simulink model "CrashAlgoSchnee_v2_analysis"  (R2020b)
settings: Solver=FixedStepAuto  StartTime=0.0  StopTime=inf  FixedStep=0.01  RelTol=1e-3
undefined symbols (not defined in the file or in its folder): magnitude
libraries: simulink x2
settings Model: Creator=snj7rt  LastModifiedBy=HNA3SI
settings DataIOCC: SaveOutput=off  SaveTime=off  ReturnWorkspaceOutputs=off
settings DebuggingCC: ArithmeticOperatorsInVariantConditions=warning
settings ModelReferenceCC: ModelReferenceNumInstancesAllowed=Single
settings SFSimCC: CustomCodeUndefinedFunction=UseInterfaceOnly
settings GRTTargetCC: CombineOutputUpdateFcns=off  MatFileLogging=off

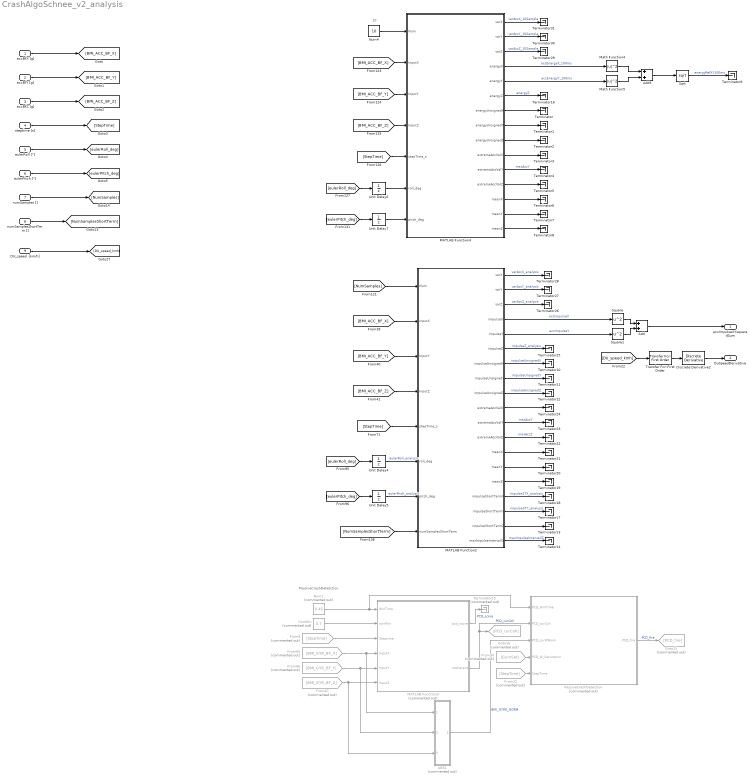
== system CrashAlgoSchnee_v2_analysis ==
  note: 10
  note: PassiveCrashDetetction
  accBfX [g] : Inport
  accBfY [g] : Inport  Port=2
  accBfZ [g] : Inport  Port=3
  steptime [s] : Inport  Port=4
  eulerRoll [°] : Inport  Port=5
  eulerPitch [°] : Inport  Port=6
  numSamples [] : Inport  Port=7
  numSamplesShortTerm [] : Inport  Port=8
  DU_speed  [km/h] : Inport  Port=9
  ABS1 : Subsystem  Commented=on
  Add : Sum
  Add3 : Sum
  CorrMin : Constant  Commented=on  Value=0.7
  Discrete Derivative2 : simulink/Discrete/Discrete Derivative  gainval=1.0  ICPrevScaledInput=0.0  OutMin=[]  OutMax=[]  OutDataType=fixdt(1, 16)  OutScaling=2^-10  DoSatur=off
  From12 : From  Commented=on  GotoTag=StepTime
  From30 : From  Commented=on  GotoTag=GyroSat
  From65 : From  Commented=on  GotoTag=BMI_GYR_BF_X
  From66 : From  Commented=on  GotoTag=BMI_GYR_BF_Y
  From67 : From  Commented=on  GotoTag=BMI_GYR_BF_Z
  From8 : From  Commented=on  GotoTag=StepTime
  Goto15 : Goto  Commented=on  GotoTag=PCD_fire
  Goto16 : Goto  Commented=on  GotoTag=PCD_curCoh
  MATLAB Function2 : MATLAB Function  TreatAsAtomicUnit=on
  MATLAB Function3 : MATLAB Function  Commented=on  TreatAsAtomicUnit=on
  MATLAB Function4 : MATLAB Function  TreatAsAtomicUnit=on
  Math Function4 : Math  Operator=magnitude^2  SignedPower=on  SaturateOnIntegerOverflow=on
  Math Function5 : Math  Operator=magnitude^2  SignedPower=on  SaturateOnIntegerOverflow=on
  Num1 : Constant  Commented=on  Value=0.45
  Num4 : Constant  Value=10
  PassiveCrashDetection : Stateflow chart  Commented=on  TreatAsAtomicUnit=on
  Sqrt : Sqrt  SaturateOnIntegerOverflow=on
  Square : Math  Operator=square  SignedPower=on  SaturateOnIntegerOverflow=on
  Square1 : Math  Operator=square  SignedPower=on  SaturateOnIntegerOverflow=on
  Terminator{,1..14,16..31} (31 alike) : Terminator
  Terminator15 : Terminator  Commented=on
  Transfer Fcn First Order : simulink/Discrete/Transfer Fcn First Order  PoleZ=0.995  ICPrevOutput=0.0  DoSatur=off
  Unit Delay{4..7} (4 alike) : UnitDelay  SampleTime=-1  HasFrameUpgradeWarning=on
  accImpulseXYsquaredSum : Outport
  DuSpeedDerivative : Outport  Port=2
  wires:
  [BMI_ACC_BF_X] -> MATLAB Function4/2(InputX)
  MATLAB Function4/3(varZ) -> Terminator29/1  "varAccZ_10Sample"
  Unit Delay7/1 -> MATLAB Function4/7(pitch_deg)
  MATLAB Function4/4(energyX) -> Math Function4/1  "accEnergyX_100ms"
  MATLAB Function4/5(energyY) -> Math Function5/1  "accEnergyY_100ms"
  MATLAB Function4/1(varX) -> Terminator31/1  "varAccX_10Sample"
  MATLAB Function4/2(varY) -> Terminator30/1  "varAccY_10Sample"
  [eulerRoll_deg] -> Unit Delay6/1
  Unit Delay6/1 -> MATLAB Function4/6(roll_deg)
  [eulerPitch_deg] -> Unit Delay7/1
  [BMI_ACC_BF_Z] -> MATLAB Function4/4(InputZ)
  Num4/1 -> MATLAB Function4/1(Num)
  [BMI_ACC_BF_Y] -> MATLAB Function4/3(InputY)
  [StepTime] -> MATLAB Function4/5(stepTime_s)
  accBfX [g]/1 -> [BMI_ACC_BF_X]
  accBfY [g]/1 -> [BMI_ACC_BF_Y]
  accBfZ [g]/1 -> [BMI_ACC_BF_Z]
  steptime [s]/1 -> [StepTime]
  eulerRoll [°]/1 -> [eulerRoll_deg]
  eulerPitch [°]/1 -> [eulerPitch_deg]
  [BMI_ACC_BF_X] -> MATLAB Function2/2(InputX)
  [StepTime] -> MATLAB Function2/5(stepTime_s)
  MATLAB Function2/17(impulseShortTermY) -> Terminator17/1  "impulseSTY_analysis"
  MATLAB Function2/7(impulseUnsignedX) -> Terminator10/1  "impulseUnsignedX"
  MATLAB Function2/19(maxImpulseIntervallZ) -> Terminator14/1  "maxImpulseIntervallZ"
  [NumSamplesShortTerm] -> MATLAB Function2/8(numSamplesShortTerm)
  [NumSamples] -> MATLAB Function2/1(Num)
  Unit Delay4/1 -> MATLAB Function2/6(roll_deg)  "eulerRoll_analysis"
  [eulerRoll_deg] -> Unit Delay4/1
  MATLAB Function2/8(impulseUnsignedY) -> Terminator11/1  "impulseUnsignedY"
  Unit Delay5/1 -> MATLAB Function2/7(pitch_deg)  "eulerPitch_analysis"
  [eulerPitch_deg] -> Unit Delay5/1
  MATLAB Function2/12(extremaAccValZ) -> Terminator22/1  "maxAccZ"
  MATLAB Function2/9(impulseUnsignedZ) -> Terminator12/1  "impulseUnsignedZ"
  MATLAB Function2/6(impulseZ) -> Terminator25/1  "impulseZ_analysis"
  MATLAB Function2/2(varY) -> Terminator27/1  "varAccY_analysis"
  MATLAB Function2/1(varX) -> Terminator28/1  "varAccX_analysis"
  MATLAB Function2/5(impulseY) -> Square1/1  "accImpulseY"
  [BMI_ACC_BF_Z] -> MATLAB Function2/4(InputZ)
  [BMI_ACC_BF_Y] -> MATLAB Function2/3(InputY)
  MATLAB Function2/4(impulseX) -> Square/1  "accImpulseX"
  MATLAB Function2/3(varZ) -> Terminator26/1  "varAccZ_analysis"
  MATLAB Function2/16(impulseShortTermX) -> Terminator18/1  "impulseSTX_analysis"
  MATLAB Function2/10(extremaAccValX) -> Terminator24/1
  MATLAB Function2/11(extremaAccValY) -> Terminator23/1  "maxAccY"
  MATLAB Function3/1(pcd_score) -> Terminator15/1  "PCD_score"
  From66/1 -> ABS1/2(In2), MATLAB Function3/5(InputY)
  From8/1 -> MATLAB Function3/3(Steptime)
  PassiveCrashDetection/1(PCD_fire) -> Goto15/1  "PCD_fire"
  From30/1 -> PassiveCrashDetection/4(PCD_W_Saturation)
  ABS1/1(Out1) -> PassiveCrashDetection/3(PCD_curWNorm)  "BMI_GYRO_NORM"
  From12/1 -> PassiveCrashDetection/5(StepTime)
  Num1/1 -> PassiveCrashDetection/1(PCD_WinTime), MATLAB Function3/1(WinTime)
  From65/1 -> ABS1/1(In1), MATLAB Function3/4(InputX)
  MATLAB Function3/2(ncoherent) -> Goto16/1, PassiveCrashDetection/2(PCD_curCoh)  "PCD_curCoh"
  From67/1 -> MATLAB Function3/6(InputZ), ABS1/3(In3)
  CorrMin/1 -> MATLAB Function3/2(corrMin)
  numSamples []/1 -> [NumSamples]
  numSamplesShortTerm []/1 -> [NumSamplesShortTerm]
  DU_speed  [km/h]/1 -> [DU_speed_kmh]
  MATLAB Function2/15(meanZ) -> Terminator19/1
  MATLAB Function2/14(meanY) -> Terminator20/1
  MATLAB Function2/13(meanX) -> Terminator21/1
  Math Function4/1 -> Add3/1
  Math Function5/1 -> Add3/2
  Add3/1 -> Sqrt/1
  Sqrt/1 -> Terminator9/1  "energyRefXY100ms"
  [DU_speed_kmh] -> Transfer Fcn First Order/1
  Discrete Derivative2/1 -> DuSpeedDerivative/1
  Transfer Fcn First Order/1 -> Discrete Derivative2/1
  MATLAB Function4/6(energyZ) -> Terminator16/1  "energyZ"
  MATLAB Function4/7(energyUnsignedX) -> Terminator/1
  MATLAB Function4/8(energyUnsignedY) -> Terminator1/1
  MATLAB Function4/9(energyUnsignedZ) -> Terminator2/1
  MATLAB Function4/10(extremaAccValX) -> Terminator3/1
  MATLAB Function4/11(extremaAccValY) -> Terminator4/1  "maxAccY"
  MATLAB Function4/12(extremaAccValZ) -> Terminator5/1
  MATLAB Function4/13(meanX) -> Terminator6/1
  MATLAB Function4/14(meanY) -> Terminator7/1
  MATLAB Function4/15(meanZ) -> Terminator8/1
  MATLAB Function2/18(impulseShortTermZ) -> Terminator13/1
  Square/1 -> Add/1
  Square1/1 -> Add/2
  Add/1 -> accImpulseXYsquaredSum/1

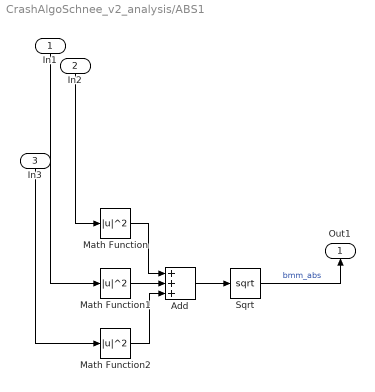
== system CrashAlgoSchnee_v2_analysis/ABS1 ==
  In1 : Inport
  In2 : Inport  Port=2
  In3 : Inport  Port=3
  Add : Sum  Inputs=+++
  Math Function : Math  Operator=magnitude^2  SignedPower=on  SaturateOnIntegerOverflow=on
  Math Function1 : Math  Operator=magnitude^2  SignedPower=on  SaturateOnIntegerOverflow=on
  Math Function2 : Math  Operator=magnitude^2  SignedPower=on  SaturateOnIntegerOverflow=on
  Sqrt : Sqrt  SaturateOnIntegerOverflow=on
  Out1 : Outport  VectorParamsAs1DForOutWhenUnconnected=off
  wires:
  In3/1 -> Math Function2/1
  In2/1 -> Math Function/1
  In1/1 -> Math Function1/1
  Math Function2/1 -> Add/3
  Add/1 -> Sqrt/1
  Math Function/1 -> Add/1
  Math Function1/1 -> Add/2
  Sqrt/1 -> Out1/1  "bmm_abs"

== matlab function CrashAlgoSchnee_v2_analysis/MATLAB Function4 ==
  data: Num input; InputX input; InputY input; InputZ input; varX output; varY output; varZ output; energyX output; energyY output; energyZ output; energyUnsignedX output; energyUnsignedY output; energyUnsignedZ output; stepTime_s input; extremaAccValX output; extremaAccValY output; roll_deg input; pitch_deg input; extremaAccValZ output; meanX output; meanY output; meanZ output
function [varX, varY, varZ, energyX, energyY, energyZ, ...
    energyUnsignedX, energyUnsignedY, energyUnsignedZ, ...
    extremaAccValX, extremaAccValY, extremaAccValZ, meanX, meanY, meanZ] = ...
    varPastNumSamples(Num, ...
    InputX, InputY, InputZ, stepTime_s, roll_deg, pitch_deg)

persistent ringBufX ringBufY ringBufZ i ringBufXgComp ringBufYgComp  
        
%% declaration only during first run!

if isempty(i)  
        ringBufX =ones(Num,1);
        ringBufY =ones(Num,1);
        ringBufYgComp =ones(Num,1);
        ringBufXgComp =ones(Num,1);
        ringBufZ =ones(Num,1);
        i = 1; 
end

ringBufX(i)= InputX;
ringBufY(i)= InputY;
ringBufYgComp(i)= InputY - sind(roll_deg);
ringBufXgComp(i)= InputX + sind(pitch_deg);
ringBufZ(i)= InputZ;

varX = var(ringBufX, 0);
varY = var(ringBufY, 0);
varZ = var(ringBufZ, 0);

if varX >= 1.5 || varY >= 1.5 || varZ >= 6 % maybe high threshold for varZ???
    %energyX = sum(ringBufX.*stepTime_s);
    energyX = sum(ringBufXgComp.*stepTime_s);
    %energyY = sum(ringBufY.*stepTime_s);
    energyY = sum(ringBufYgComp.*stepTime_s);
    energyZ = sum(ringBufZ.*stepTime_s); 
    energyUnsignedX = sum(abs(ringBufX).*stepTime_s);
    energyUnsignedY = sum(abs(ringBufY).*stepTime_s); 
    energyUnsignedZ = sum(abs(ringBufZ).*stepTime_s); 
else
%     energyX = 0;
%     energyY = 0; 
%     energyZ = 0;
    %energyX = sum(ringBufX.*stepTime_s);
    energyX = sum(ringBufXgComp.*stepTime_s);
    %energyY = sum(ringBufY.*stepTime_s);
    energyY = sum(ringBufYgComp.*stepTime_s);
    energyZ = sum(ringBufZ.*stepTime_s); 
    energyUnsignedX = 0;
    energyUnsignedY = 0; 
    energyUnsignedZ = 0; 
end

extremaAccValX = max(abs(ringBufX));
%extremaAccValY = max(abs(ringBufY));
extremaAccValZ = max(abs(ringBufZ));

[extremaAccValY, extremaIndY] = max(abs(ringBufY));
if sign(ringBufY(extremaIndY)) == 1
    %extremaAccValY = extremaAccValY;
else
    extremaAccValY = extremaAccValY * -1;
end

meanX = mean(ringBufXgComp);
meanY = mean(ringBufYgComp);
meanZ = mean(ringBufZ);

i = i +1;
if i > Num
    i = 1;
end

== matlab function CrashAlgoSchnee_v2_analysis/MATLAB Function2 ==
  data: Num input; InputX input; InputY input; InputZ input; varX output; varY output; varZ output; impulseX output; impulseY output; impulseZ output; impulseUnsignedX output; impulseUnsignedY output; impulseUnsignedZ output; extremaAccValX output; stepTime_s input; extremaAccValY output; extremaAccValZ output; meanX output; meanY output; meanZ output; roll_deg input; pitch_deg input; numSamplesShortTerm input; impulseShortTermX output; impulseShortTermY output; impulseShortTermZ output; maxImpulseIntervallZ output
function [varX, varY, varZ, impulseX, impulseY, impulseZ, ...
    impulseUnsignedX, impulseUnsignedY, impulseUnsignedZ, ...
    extremaAccValX, extremaAccValY, extremaAccValZ, meanX, meanY, meanZ, ...
    impulseShortTermX, impulseShortTermY, impulseShortTermZ, maxImpulseIntervallZ] = ...
    varPastNumSamples(Num, ...
    InputX, InputY, InputZ, stepTime_s, roll_deg, pitch_deg, numSamplesShortTerm)

gCompensation = 1;

persistent ringBufX ringBufY ringBufZ i ringBufXgComp ringBufYgComp ...
    ringBufZgComp ringBufmaxImpulseZ NumlatchedImpulseZ b
        
%% declaration only during first run!

if isempty(i)  
        NumlatchedImpulseZ = 10;
        ringBufX = zeros(Num,1);
        ringBufY = zeros(Num,1);
        ringBufZ = zeros(Num,1);
        ringBufYgComp = zeros(Num,1);
        ringBufXgComp = zeros(Num,1);
        ringBufZgComp = zeros(Num,1);
        ringBufmaxImpulseZ = zeros(NumlatchedImpulseZ,1);
        i = 1; 
        b = 1;
end

ringBufX(i) = InputX;
ringBufY(i) = InputY;
ringBufZ(i) = InputZ;
ringBufXgComp(i) = InputX + sind(pitch_deg);
ringBufYgComp(i) = InputY - sind(roll_deg);
ringBufZgComp(i) = InputZ - cosd(pitch_deg);


varX = var(ringBufX, 0);
varY = var(ringBufY, 0);
varZ = var(ringBufZ, 0);

% indicesMutedLatchedImpulseZ = b-4:b;
% 
% for a=1:length(indicesMutedLatchedImpulseZ)
%     if indicesMutedLatchedImpulseZ(a) <= 0
%         indicesMutedLatchedImpulseZ(a) = indicesMutedLatchedImpulseZ(a)+ NumlatchedImpulseZ;
%     end
% end

indicesShortTerm = i-(numSamplesShortTerm-1):i;
for a=1:length(indicesShortTerm)
    if indicesShortTerm(a) <= 0
        indicesShortTerm(a) = indicesShortTerm(a)+ Num;
    end
end


% if varX >= 1.5 || varY >= 1.5 || varZ >= 6 % maybe high threshold for varZ???
%     impulseUnsignedX = sum(abs(ringBufX).*stepTime_s);
%     impulseUnsignedY = sum(abs(ringBufY).*stepTime_s); 
%     impulseUnsignedZ = sum(abs(ringBufZ).*stepTime_s); 
% else
%     impulseUnsignedX = 0;
%     impulseUnsignedY = 0; 
%     impulseUnsignedZ = 0; 
% end

if  gCompensation == 1
    impulseX = sum(ringBufXgComp.*stepTime_s);
    impulseY = sum(ringBufYgComp.*stepTime_s);
    impulseZ = sum(ringBufZgComp.*stepTime_s);
    impulseShortTermX = sum(ringBufXgComp(indicesShortTerm).*stepTime_s);
    impulseShortTermY = sum(ringBufYgComp(indicesShortTerm).*stepTime_s);
    impulseShortTermZ = sum(ringBufZ(indicesShortTerm).*stepTime_s);
    meanX = mean(ringBufXgComp);
    meanY = mean(ringBufYgComp);
    meanZ = mean(ringBufZgComp);
else
    impulseX = sum(ringBufX.*stepTime_s);
    impulseY = sum(ringBufY.*stepTime_s);
    impulseZ = sum(ringBufZ.*stepTime_s);
    impulseShortTermX = sum(ringBufX(indicesShortTerm).*stepTime_s);
    impulseShortTermY = sum(ringBufY(indicesShortTerm).*stepTime_s);
    impulseShortTermZ = sum(ringBufZ(indicesShortTerm).*stepTime_s);
    meanX = mean(ringBufX);
    meanY = mean(ringBufY);
    meanZ = mean(ringBufZ);
end

ringBufmaxImpulseZ(b) = impulseZ;
maxImpulseIntervallZ = max(abs(ringBufmaxImpulseZ));

impulseUnsignedX = sum(abs(ringBufX).*stepTime_s);
impulseUnsignedY = sum(abs(ringBufY).*stepTime_s); 
impulseUnsignedZ = sum(abs(ringBufZ).*stepTime_s); 

extremaAccValX = max(abs(ringBufX));
%extremaAccValY = max(abs(ringBufY));
extremaAccValZ = max(abs(ringBufZ));

[extremaAccValY, extremaIndY] = max(abs(ringBufY));
if sign(ringBufY(extremaIndY)) == 1
    %extremaAccValY = extremaAccValY;
else
    extremaAccValY = extremaAccValY * -1;
end



i = i + 1;
if i > Num
    i = 1;
end

b = b + 1;
if b > NumlatchedImpulseZ
    b = 1;
end

== matlab function CrashAlgoSchnee_v2_analysis/MATLAB Function3 ==
  data: WinTime input; corrMin input; Steptime input; InputX input; InputY input; InputZ input; pcd_score output; ncoherent output
function [pcd_score, ncoherent] = dotProdPastNumSamples(WinTime,corrMin, Steptime,InputX,InputY,InputZ)

persistent ringBuf i Num gyroNormedRingBuf
        
%% declaration only during first run!
if isempty(i)
        Num = floor(WinTime * 1/Steptime);
        ringBuf =ones(Num,3);        
        i = 1;
        gyroNormedRingBuf = ones(Num,3);
end

%%

ringBuf(i,1)= InputX;
ringBuf(i,2)= InputY;
ringBuf(i,3)= InputZ;

%normalized in order to calculate mutual dot product

gyroNormedRingBuf(i,:) = ringBuf(i,:)./(sqrt(ringBuf(i,1)^2 + ringBuf(i,2)^2 + ringBuf(i,3)^2));

%calculate mutual dot product
g_corr =  gyroNormedRingBuf * gyroNormedRingBuf.';

pcd_score = min(min(g_corr));
ncoherent = sum(sum(g_corr > corrMin));

i = i +1;
if i > Num
    i = 1;
end

== stateflow chart CrashAlgoSchnee_v2_analysis/PassiveCrashDetection ==
  state Init
    en:
    PCD_LATCHTIME = 5;  %sec
    PCD_SLEEPTIME = 4;  %sec
    %PCD_W_MIN = 3;   %min rotational rate
    PCD_W_MIN = 80;   %min rotational rate
    PCD_CohThresh = (1/StepTime * PCD_WinTime)^2;
    PCD_fire = 0;
  state CheckWNorm
    en:
    PCD_fire = 0;
  state G_Saturation
  state CheckForUnforcedTipover
  state Sleep
  state Latch
  (default) -> Init
  Init -> CheckWNorm : [after(PCD_WinTime,sec)]
      | %wait for ringbuffer
  Sleep -> CheckWNorm : [after(PCD_SLEEPTIME,sec)]
  Latch -> CheckWNorm : [after(PCD_LATCHTIME,sec)]
  G_Saturation -> CheckWNorm : [after(PCD_WinTime,sec)]
  CheckWNorm -> CheckForUnforcedTipover : [PCD_curWNorm >= PCD_W_MIN]
  CheckForUnforcedTipover -> G_Saturation [order 1] : [PCD_W_Saturation==1]
  CheckForUnforcedTipover -> Sleep [order 2] : [PCD_curCoh <PCD_CohThresh]
  CheckForUnforcedTipover -> Latch [order 3] : [PCD_curCoh >=PCD_CohThresh]
      | {
      | PCD_fire = 1;
      | }
  data: PCD_WinTime input; PCD_curCoh input; PCD_curWNorm input; PCD_W_Saturation input; StepTime input; PCD_SLEEPTIME local; PCD_fire output; PCD_CohThresh local; PCD_LATCHTIME local; PCD_W_MIN local
